simulink model "SimuRampaContinuo"  (R2020a)
settings: Solver=VariableStepAuto  StartTime=0.0  StopTime=3  RelTol=1e-3
undefined symbols (not defined in the file): kd1, kd2, ki1, ki2, kp, mu, tm
libraries: simulink x2
settings Model: Creator=Alexander  LastModifiedBy=AsusPC
settings DataIOCC: ReturnWorkspaceOutputs=off
settings DebuggingCC: ArithmeticOperatorsInVariantConditions=warning
settings SFSimCC: SimUseLocalCustomCode=off  CustomCodeUndefinedFunction=UseInterfaceOnly
settings RTWCC: RTWUseLocalCustomCode=off

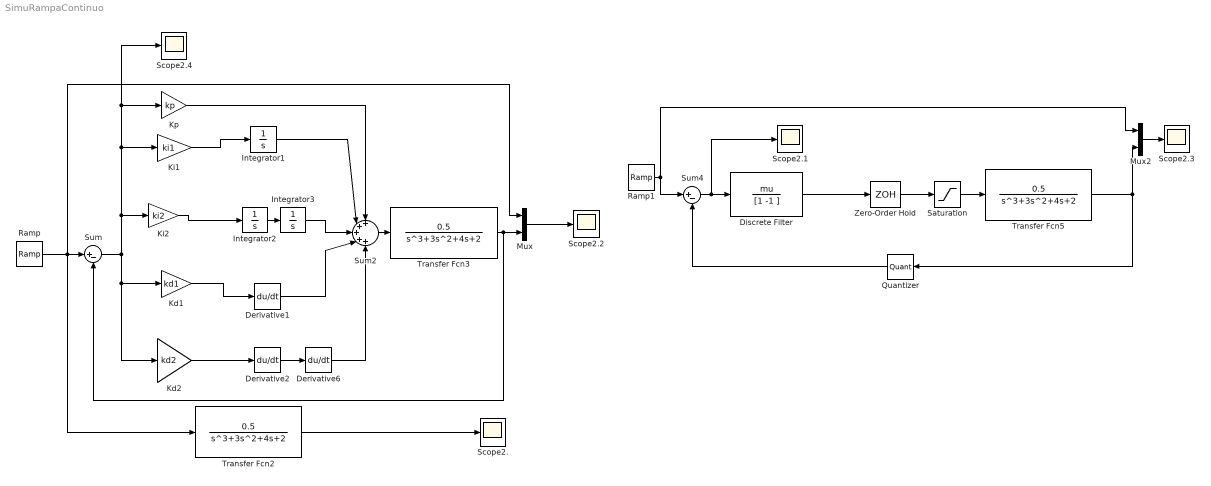
== system SimuRampaContinuo ==
  Derivative1 : Derivative
  Derivative2 : Derivative
  Derivative6 : Derivative
  Discrete Filter : DiscreteFilter  Numerator=mu  Denominator=[1 -1 ]  SampleTime=tm
  Integrator1 : Integrator
  Integrator2 : Integrator
  Integrator3 : Integrator
  Kd1 : Gain  Gain=kd1
  Kd2 : Gain  Gain=kd2
  Ki1 : Gain  Gain=ki1
  Ki2 : Gain  Gain=ki2
  Kp : Gain  Gain=kp
  Mux : Mux  Inputs=2
  Mux2 : Mux  Inputs=2
  Quantizer : Quantizer  QuantizationInterval=3.3/1024
  Ramp : simulink/Sources/Ramp  slope=1  start=0.1  InitialOutput=0
  Ramp1 : simulink/Sources/Ramp  slope=1  start=0  InitialOutput=0
  Saturation : Saturate  UpperLimit=70  LowerLimit=-70
  Scope2.{,1..4} (5 alike) : Scope
  Sum : Sum  Inputs=|+-
  Sum2 : Sum  Inputs=+++++
  Sum4 : Sum  Inputs=|+-
  Transfer Fcn2 : TransferFcn  Numerator=[0.5]  Denominator=[1 3 4 2]
  Transfer Fcn3 : TransferFcn  Numerator=[0.5]  Denominator=[1 3 4 2]
  Transfer Fcn5 : TransferFcn  Numerator=[0.5]  Denominator=[1 3 4 2]
  Zero-Order Hold : ZeroOrderHold  SampleTime=tm
  wires:
  Sum2/1 -> Transfer Fcn3/1
  Transfer Fcn3/1 -> Mux/2, Sum/2
  Sum/1 -> Scope2.4/1, Kp/1, Ki1/1, Ki2/1, Kd2/1, Kd1/1
  Kd2/1 -> Derivative2/1
  Ki1/1 -> Integrator1/1
  Derivative2/1 -> Derivative6/1
  Kd1/1 -> Derivative1/1
  Integrator1/1 -> Sum2/2
  Transfer Fcn2/1 -> Scope2./1
  Kp/1 -> Sum2/1
  Ramp/1 -> Mux/1, Sum/1, Transfer Fcn2/1
  Mux/1 -> Scope2.2/1
  Integrator2/1 -> Integrator3/1
  Ki2/1 -> Integrator2/1
  Integrator3/1 -> Sum2/3
  Derivative1/1 -> Sum2/4
  Derivative6/1 -> Sum2/5
  Saturation/1 -> Transfer Fcn5/1
  Ramp1/1 -> Mux2/1, Sum4/1
  Mux2/1 -> Scope2.3/1
  Zero-Order Hold/1 -> Saturation/1
  Discrete Filter/1 -> Zero-Order Hold/1
  Sum4/1 -> Scope2.1/1, Discrete Filter/1
  Transfer Fcn5/1 -> Quantizer/1, Mux2/2
  Quantizer/1 -> Sum4/2
